simulink library "RoboticsCode"  (R2023a)
settings: Solver=VariableStepAuto  StartTime=0.0  StopTime=10.0  RelTol=1e-3
undefined symbols (not defined in the file or in its folder): SampleTime
settings Model: Creator=kgross  LastModifiedBy=kgross
settings SFSimCC: SimCustomHeaderCode="#include \"kinematics.h\""  SimCustomInitializer=initializeMemory();  SimCustomTerminator=freeMemory();  SimUserIncludeDirs=../include  SimUserLibraries=lib/kinematics.lib  SimTargetLang=C++

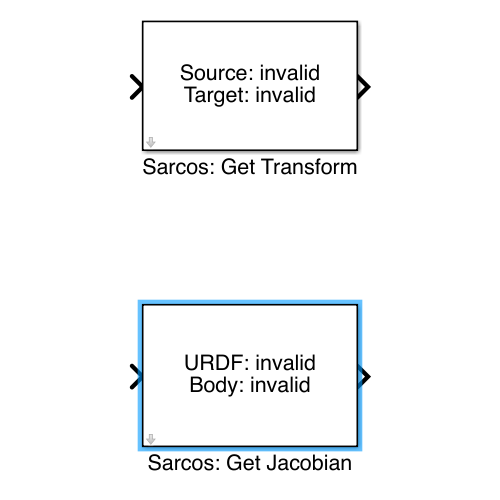
[thumbnail: Simulink's stored preview of the top-level diagram]
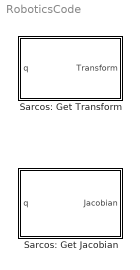
== system RoboticsCode ==
  Sarcos: Get Jacobian : Subsystem  StartFcn=assignin('base', 'MaskWorkspace', 'base');  StopFcn=evalin('base', 'clear MaskWorkspace');  mask{urdfpath='invalid', source=invalid, source_string='invalid'}
      mask prompts: urdfpath "URDF:"; source "Body:"
      mask TypeOptions source: invalid
      mask DialogControl browsebutton Prompt: Browse
      mask Display:
      | thisUrdf = get_param(gcb, "urdfpath");
      | thisUrdf = evalin('base', thisUrdf);
      | thisUrdf = strsplit(thisUrdf, "/");
      | thisUrdf = strsplit(thisUrdf{end}, "\");
      | thisUrdf = thisUrdf{end};
      | 
      | thisBody = get_param(gcb, "source");
      | fprintf("URDF: %s\nBody: %s", strrep(thisUrdf, "'", ""), strrep(thisBody, "'", ""));
  Sarcos: Get Transform : Subsystem  mask{urdfpath='invalid', source=invalid, source_string='invalid', target=invalid, target_string='invalid'}
      mask prompts: urdfpath "URDF:"
      mask TypeOptions source: invalid
      mask TypeOptions target: invalid
      mask DialogControl browsebutton Prompt: Browse
      mask Display:
      | thisSource = get_param(gcb, "source");
      | thisTarget = get_param(gcb, "target");
      | 
      | fprintf("Source: %s\nTarget: %s", thisSource, thisTarget);

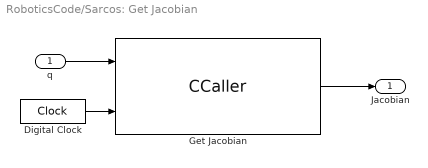
== system RoboticsCode/Sarcos: Get Jacobian ==
  q : Inport
  Digital Clock : DigitalClock
  Get Jacobian : CCaller  FunctionName=GetJacobianForBody  PortSpecificationStruct="%)30     .    N H   8    (     @         %    \"     8    !     0         %  0 \"0    $    _    07)G3F%M90  4&]R=$YA;64 4V-O<&4     26YD97@     5'EP90      4VEZ90      27-';&]B86P   X    X    !@    @    $          4    (     0    @    !         !     (    =7)D9G!A=&@.    .     8    (    !          %    \"     $    (     0         0    \"    '5R9&9P871H#@   $     &    \"     0         !0    @    !  ...(+3322 chars)"  SampleTime=SampleTime  urdfpath=uint8(which(urdfpath))  urdflen=length(which(urdfpath))  bodyName=uint8(source_string)  SampleTime=-1
  Jacobian : Outport
  wires:
  q/1 -> Get Jacobian/1
  Get Jacobian/1 -> Jacobian/1
  Digital Clock/1 -> Get Jacobian/2

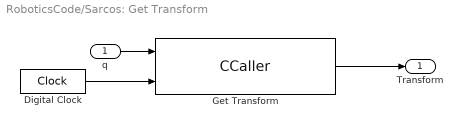
== system RoboticsCode/Sarcos: Get Transform ==
  q : Inport
  Digital Clock : DigitalClock
  Get Transform : CCaller  FunctionName=TransformFromTo  PortSpecificationStruct="%)30     .    @ P   8    (     @         %    \"     <    !     0         %  0 \"0    $    _    07)G3F%M90  4&]R=$YA;64 4V-O<&4     26YD97@     5'EP90      4VEZ90      27-';&]B86P   X    X    !@    @    $          4    (     0    @    !         !     (    =7)D9G!A=&@.    .     8    (    !          %    \"     $    (     0         0    \"    '5R9&9P871H#@   $     &    \"     0         !0    @    !  ...(+3938 chars)"  SampleTime=SampleTime  urdfpath=uint8(which(urdfpath))  urdflen=length(which(urdfpath))  source=uint8(source_string)  target=uint8(target_string)  SampleTime=-1
  Transform : Outport
  wires:
  q/1 -> Get Transform/1
  Digital Clock/1 -> Get Transform/2
  Get Transform/1 -> Transform/1
